simulink model "Competencia"  (R2021b)
settings: Solver=VariableStepAuto  StartTime=0.0  StopTime=10.0  RelTol=1e-3
undefined symbols (not defined in the file): alpha12, alpha21, k1, k2, N10, N20, r1, r2
settings Model: Creator=curie  LastModifiedBy=alex
settings SolverCC: AlgebraicLoopSolver=TrustRegion
settings DebuggingCC: SFMachineParentedDataDiag=warning

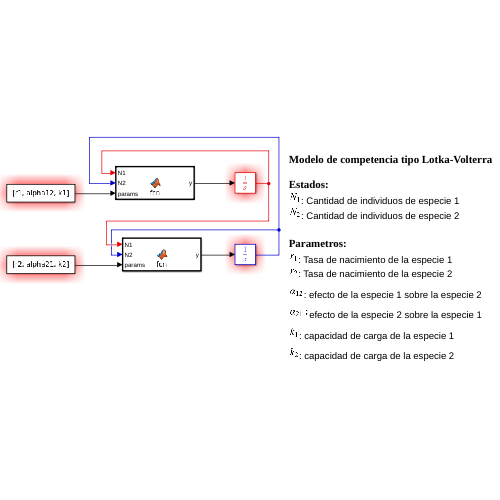
[thumbnail: Simulink's stored preview of the top-level diagram]
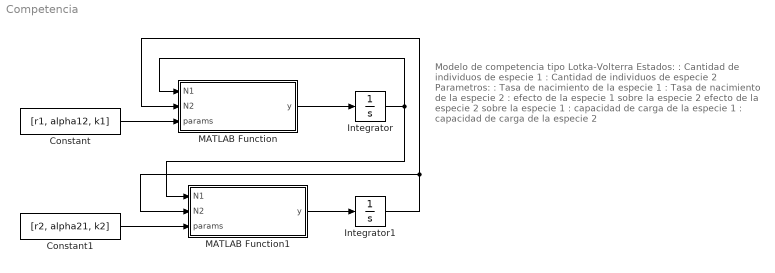
== system Competencia ==
  note: Modelo de competencia tipo Lotka-Volterra
      |
      | Estados:
      | : Cantidad de individuos de especie 1
      | : Cantidad de individuos de especie 2
      |
      | Parametros:
      | : Tasa de nacimiento de la especie 1
      | : Tasa de nacimiento de la especie 2
      | : efecto de la especie 1 sobre la especie 2
      | efecto de la especie 2 sobre la especie 1
      | : capacidad de carga de la especie 1
      | : capacidad de carga de la especie 2
  Constant : Constant  Value=[r1, alpha12, k1]
  Constant1 : Constant  Value=[r2, alpha21, k2]
  Integrator : Integrator  InitialCondition=N10
  Integrator1 : Integrator  InitialCondition=N20
  MATLAB Function : MATLAB Function  TreatAsAtomicUnit=on
  MATLAB Function1 : MATLAB Function  TreatAsAtomicUnit=on
  wires:
  MATLAB Function/1(y) -> Integrator/1
  MATLAB Function1/1(y) -> Integrator1/1
  Integrator/1 -> MATLAB Function/1(N1), MATLAB Function1/1(N1)
  Integrator1/1 -> MATLAB Function1/2(N2), MATLAB Function/2(N2)
  Constant/1 -> MATLAB Function/3(params)
  Constant1/1 -> MATLAB Function1/3(params)

== matlab function Competencia/MATLAB Function ==
  data: N1 input; y output; N2 input; params input
function y = fcn(N1, N2, params)

r1 = params(1);
alpha12 = params(2);
k1 = params(3);

y = r1*N1*(1-(N1+alpha12*N2)/k1);

== matlab function Competencia/MATLAB Function1 ==
  data: N1 input; y output; N2 input; params input
function y = fcn(N1, N2, params)

r2 = params(1);
alpha21 = params(2);
k2 = params(3);

y = r2*N2*(1-(N2+alpha21*N1)/k2);
